simulink model "CAN"  (R2020a)
settings: Solver=FixedStepAuto  StartTime=0.0  StopTime=10.0  RelTol=1e-3
libraries: canmsglib x5
settings Model: Creator=10661011  LastModifiedBy=99661217
settings OptimizationCC: DefaultParameterBehavior=Inlined  EnhancedBackFolding=on  PassReuseOutputArgsAs=Individual arguments  ZeroExternalMemoryAtStartup=off  ZeroInternalMemoryAtStartup=off  OptimizeBlockOrder=speed  DifferentSizesBufferReuse=on  OptimizationCustomize=off  EfficientTunableParamExpr=on
settings DebuggingCC: ParameterTunabilityLossMsg=error
settings HardwareCC: ProdBitPerInt=16  ProdBitPerPointer=8  ProdBitPerSizeT=24  ProdBitPerPtrDiffT=24  ProdLargestAtomicFloat=None  ProdWordSize=8  ProdHWDeviceType=Microchip->PIC18
settings SFSimCC: MATLABDynamicMemAlloc=off
settings RTWCC: SystemTargetFile=ert.tlc  TemplateMakefile=ert_default_tmf
settings CodeAppCC: ForceParamTrailComments=on  IgnoreCustomStorageClasses=off  OperatorAnnotations=on  SimulinkDataObjDesc=on  SFDataObjDesc=on  InsertBlockDesc=on
settings ERTTargetCC: TargetLangStandard=C99 (ISO)  GenerateSampleERTMain=on  InlinedParameterPlacement=NonHierarchical  ERTCustomFileTemplate=example_file_process.tlc

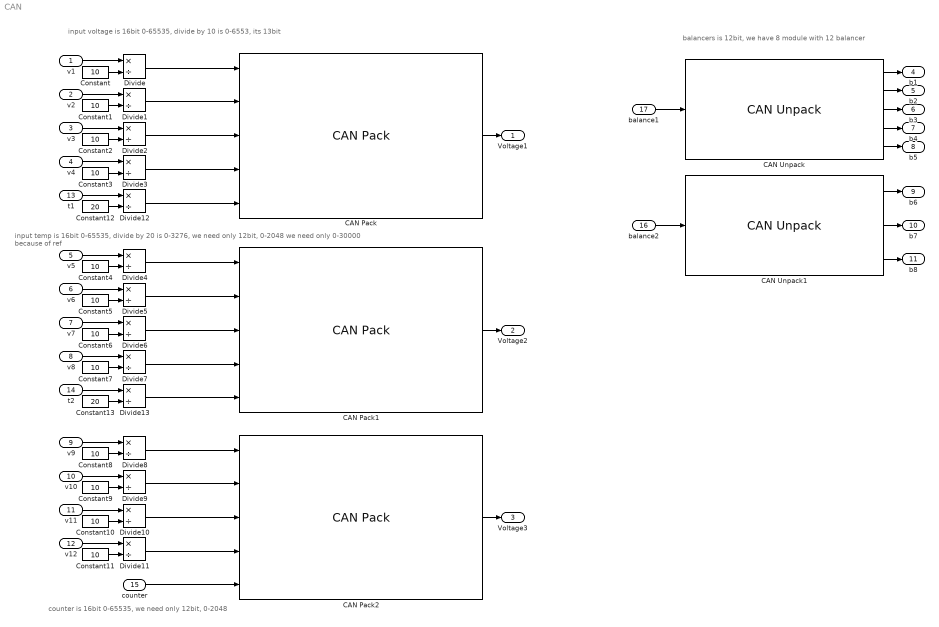
== system CAN ==
  note: input voltage is 16bit 0-65535, divide by 10 is 0-6553, its 13bit
  note: input temp is 16bit 0-65535, divide by 20 is 0-3276, we need only 12bit, 0-2048 we need only 0-30000 because of ref
  note: counter is 16bit 0-65535, we need only 12bit, 0-2048
  note: balancers is 12bit, we have 8 module with 12 balancer
  v1 : Inport  OutDataTypeStr=uint16
  v2 : Inport  Port=2  OutDataTypeStr=uint16
  v3 : Inport  Port=3  OutDataTypeStr=uint16
  v4 : Inport  Port=4  OutDataTypeStr=uint16
  v5 : Inport  Port=5  OutDataTypeStr=uint16
  v6 : Inport  Port=6  OutDataTypeStr=uint16
  v7 : Inport  Port=7  OutDataTypeStr=uint16
  v8 : Inport  Port=8  OutDataTypeStr=uint16
  v9 : Inport  Port=9  OutDataTypeStr=uint16
  v10 : Inport  Port=10  OutDataTypeStr=uint16
  v11 : Inport  Port=11  OutDataTypeStr=uint16
  v12 : Inport  Port=12  OutDataTypeStr=uint16
  t1 : Inport  Port=13  OutDataTypeStr=uint16
  t2 : Inport  Port=14  OutDataTypeStr=uint16
  counter : Inport  Port=15  OutDataTypeStr=uint16
  balance2 : Inport  Port=16  OutDataTypeStr=Bus: CAN_MESSAGE_BUS  BusOutputAsStruct=on
  balance1 : Inport  Port=17  OutDataTypeStr=Bus: CAN_MESSAGE_BUS  BusOutputAsStruct=on
  CAN Pack : canmsglib/CAN Pack  MsgList=(none)  MsgName=CellData1  MsgIDType=Standard (11-bit identifier)  MsgIdentifier=0  MsgLength=8  Remote=off  ApplyMinMax=off  BusOutput=on  SignalInfo={ 'v1', '0', '13', 'LE', 'unsigned', 'Standard', '0', '1', '0', '0', 'inf'; 'v2', '13', '13', 'LE', 'unsigned', 'Standard', '0', '1', '0', '0', 'inf'; 'v3', '26', '13', 'LE', 'unsigned', 'Standard', '0', '1', '0', '0', 'inf'; 'v4', '39', '13', 'LE', 'unsigned', 'Standard', '0', '1', '0', '0', 'inf'; 't1', '52', '12', 'LE', 'unsigned', 'Standard', '0', '1', '0', '0', 'inf' }
      settings: SourceProductBaseCode=ME,VN  DataFormat=manually specified signals
  CAN Pack1 : canmsglib/CAN Pack  MsgList=(none)  MsgName=CellData2  MsgIDType=Standard (11-bit identifier)  MsgIdentifier=0  MsgLength=8  Remote=off  ApplyMinMax=off  BusOutput=on  SignalInfo={ 'v5', '0', '13', 'LE', 'unsigned', 'Standard', '0', '1', '0', '0', 'inf'; 'v6', '13', '13', 'LE', 'unsigned', 'Standard', '0', '1', '0', '0', 'inf'; 'v7', '26', '13', 'LE', 'unsigned', 'Standard', '0', '1', '0', '0', 'inf'; 'v8', '39', '13', 'LE', 'unsigned', 'Standard', '0', '1', '0', '0', 'inf'; 't2', '52', '12', 'LE', 'unsigned', 'Standard', '0', '1', '0', '0', 'inf' }
      settings: SourceProductBaseCode=ME,VN  DataFormat=manually specified signals
  CAN Pack2 : canmsglib/CAN Pack  MsgList=(none)  MsgName=CellData3  MsgIDType=Standard (11-bit identifier)  MsgIdentifier=0  MsgLength=8  Remote=off  ApplyMinMax=off  BusOutput=on  SignalInfo={ 'v9', '0', '13', 'LE', 'unsigned', 'Standard', '0', '1', '0', '0', 'inf'; 'v10', '13', '13', 'LE', 'unsigned', 'Standard', '0', '1', '0', '0', 'inf'; 'v11', '26', '13', 'LE', 'unsigned', 'Standard', '0', '1', '0', '0', 'inf'; 'v12', '39', '13', 'LE', 'unsigned', 'Standard', '0', '1', '0', '0', 'inf'; 'counter', '52', '12', 'LE', 'unsigned', 'Standard', '0', '1', '0', '0', 'inf' }
      settings: SourceProductBaseCode=ME,VN  DataFormat=manually specified signals
  CAN Unpack : canmsglib/CAN Unpack  MsgList=(none)  MsgName=Balance1  MsgIDType=Standard (11-bit identifier)  MsgIdentifier=1  MsgLength=8  SignalInfo={ 'b1', '0', '12', 'LE', 'unsigned', 'Standard', '0', '1', '0', '0', 'Inf'; 'b2', '12', '12', 'LE', 'unsigned', 'Standard', '0', '1', '0', '0', 'Inf'; 'b3', '24', '12', 'LE', 'unsigned', 'Standard', '0', '1', '0', '0', 'Inf'; 'b4', '36', '12', 'LE', 'unsigned', 'Standard', '0', '1', '0', '0', 'Inf'; 'b5', '48', '12', 'LE', 'unsigned', 'Standard', '0', '1', '0', '0', 'Inf' }  IDPort=off  TimestampPort=off  ErrorPort=off  RemotePort=off  LengthPort=off  StatusPort=off  ApplyMinMax=off
      settings: SourceProductBaseCode=ME,VN
  CAN Unpack1 : canmsglib/CAN Unpack  MsgList=(none)  MsgName=Balance2  MsgIDType=Standard (11-bit identifier)  MsgIdentifier=2  MsgLength=8  SignalInfo={ 'b6', '0', '12', 'LE', 'unsigned', 'Standard', '0', '1', '0', '0', 'Inf'; 'b7', '12', '12', 'LE', 'unsigned', 'Standard', '0', '1', '0', '0', 'Inf'; 'b8', '24', '12', 'LE', 'unsigned', 'Standard', '0', '1', '0', '0', 'Inf' }  IDPort=off  TimestampPort=off  ErrorPort=off  RemotePort=off  LengthPort=off  StatusPort=off  ApplyMinMax=off
      settings: SourceProductBaseCode=ME,VN
  Constant{,1..11} (12 alike) : Constant  Value=10  OutDataTypeStr=uint8
  Constant12 : Constant  Value=20  OutDataTypeStr=uint8
  Constant13 : Constant  Value=20  OutDataTypeStr=uint8
  Divide{,1..13} (14 alike) : Product  Inputs=*/  OutDataTypeStr=uint16
  Voltage1 : Outport  OutDataTypeStr=Bus: CAN_MESSAGE_BUS  BusOutputAsStruct=on
  Voltage2 : Outport  Port=2  OutDataTypeStr=Bus: CAN_MESSAGE_BUS
  Voltage3 : Outport  Port=3  OutDataTypeStr=Bus: CAN_MESSAGE_BUS
  b1 : Outport  Port=4  OutDataTypeStr=uint16
  b2 : Outport  Port=5  OutDataTypeStr=uint16
  b3 : Outport  Port=6  OutDataTypeStr=uint16
  b4 : Outport  Port=7  OutDataTypeStr=uint16
  b5 : Outport  Port=8  OutDataTypeStr=uint16
  b6 : Outport  Port=9  OutDataTypeStr=uint16
  b7 : Outport  Port=10  OutDataTypeStr=uint16
  b8 : Outport  Port=11  OutDataTypeStr=uint16
  wires:
  CAN Pack/1 -> Voltage1/1
  balance1/1 -> CAN Unpack/1
  v1/1 -> Divide/1
  Constant/1 -> Divide/2
  CAN Pack1/1 -> Voltage2/1
  CAN Pack2/1 -> Voltage3/1
  v2/1 -> Divide1/1
  Constant1/1 -> Divide1/2
  Divide1/1 -> CAN Pack/2
  Constant2/1 -> Divide2/2
  v3/1 -> Divide2/1
  Divide2/1 -> CAN Pack/3
  v4/1 -> Divide3/1
  Constant3/1 -> Divide3/2
  Divide3/1 -> CAN Pack/4
  v5/1 -> Divide4/1
  Constant4/1 -> Divide4/2
  Divide4/1 -> CAN Pack1/1
  v6/1 -> Divide5/1
  Constant5/1 -> Divide5/2
  Divide5/1 -> CAN Pack1/2
  v7/1 -> Divide6/1
  Constant6/1 -> Divide6/2
  Divide6/1 -> CAN Pack1/3
  v8/1 -> Divide7/1
  Constant7/1 -> Divide7/2
  Divide7/1 -> CAN Pack1/4
  v9/1 -> Divide8/1
  Constant8/1 -> Divide8/2
  Divide8/1 -> CAN Pack2/1
  v10/1 -> Divide9/1
  Constant9/1 -> Divide9/2
  Divide9/1 -> CAN Pack2/2
  v11/1 -> Divide10/1
  Constant10/1 -> Divide10/2
  Divide10/1 -> CAN Pack2/3
  v12/1 -> Divide11/1
  Constant11/1 -> Divide11/2
  Divide11/1 -> CAN Pack2/4
  t1/1 -> Divide12/1
  Constant12/1 -> Divide12/2
  Divide12/1 -> CAN Pack/5
  t2/1 -> Divide13/1
  Constant13/1 -> Divide13/2
  Divide13/1 -> CAN Pack1/5
  counter/1 -> CAN Pack2/5
  balance2/1 -> CAN Unpack1/1
  CAN Unpack/1 -> b1/1
  CAN Unpack/2 -> b2/1
  CAN Unpack/3 -> b3/1
  CAN Unpack/4 -> b4/1
  CAN Unpack/5 -> b5/1
  CAN Unpack1/1 -> b6/1
  CAN Unpack1/2 -> b7/1
  CAN Unpack1/3 -> b8/1
  Divide/1 -> CAN Pack/1
